simulink model "modelo_nlinear_iris"  (R2016a)
settings: Solver=ode1  StartTime=0.0  StopTime=25  FixedStep=0.01  RelTol=1e-3
undefined symbols (not defined in the file): Regions
settings Model: Creator=schul  LastModifiedBy=schul

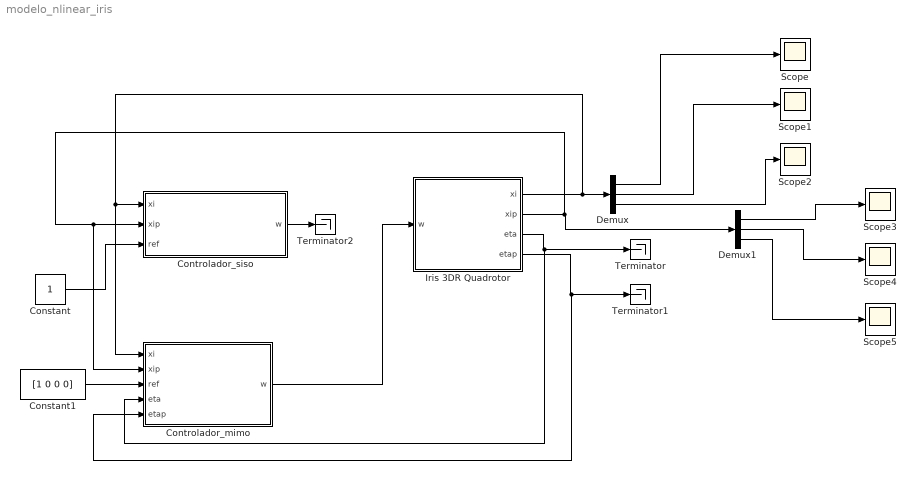
== system modelo_nlinear_iris ==
  Constant : Constant
  Constant1 : Constant  Value=[1 0 0 0]
  Controlador_mimo : Subsystem  mask{g=9.81, m=1.37, KT=15.67e-6, KD=2.551e-7, lx=0.13, ly=0.21, Ir=2.5206e-10, Ixx=0.0219, Iyy=0.0109, Izz=0.0306, Ax=0.25, Ay=0.25, Az=0.25}
  Controlador_siso : Subsystem  mask{g=9.81, m=1.37, KT=15.67e-6, KD=2.551e-7, lx=0.13, ly=0.21, Ir=2.5206e-10, Ixx=0.0219, Iyy=0.0109, Izz=0.0306, Ax=0.25, Ay=0.25, Az=0.25, Regions=Regions}
  Demux : Demux  Outputs=3
  Demux1 : Demux  Outputs=3
  Iris 3DR Quadrotor : Subsystem  mask{g=9.81, m=1.37, KT=15.67e-6, KD=2.551e-7, lx=0.13, ly=0.21, Ir=2.5206e-10, Ixx=0.0219, Iyy=0.0109, Izz=0.0306, Ax=0.25, Ay=0.25, Az=0.25}
  Scope{,1..5} (6 alike) : Scope
  Terminator : Terminator
  Terminator1 : Terminator
  Terminator2 : Terminator
  wires:
  Demux/1 -> Scope/1
  Demux/2 -> Scope1/1
  Demux/3 -> Scope2/1
  Demux1/1 -> Scope3/1
  Demux1/2 -> Scope4/1
  Demux1/3 -> Scope5/1
  Iris 3DR Quadrotor/1(xi) -> Controlador_mimo/1(xi), Controlador_siso/1(xi), Demux/1
  Iris 3DR Quadrotor/2(xip) -> Controlador_mimo/2(xip), Controlador_siso/2(xip), Demux1/1
  Constant/1 -> Controlador_siso/3(ref)
  Constant1/1 -> Controlador_mimo/3(ref)
  Iris 3DR Quadrotor/4(etap) -> Controlador_mimo/5(etap), Terminator1/1
  Iris 3DR Quadrotor/3(eta) -> Controlador_mimo/4(eta), Terminator/1
  Controlador_siso/1(w) -> Terminator2/1
  Controlador_mimo/1(w) -> Iris 3DR Quadrotor/1(w)

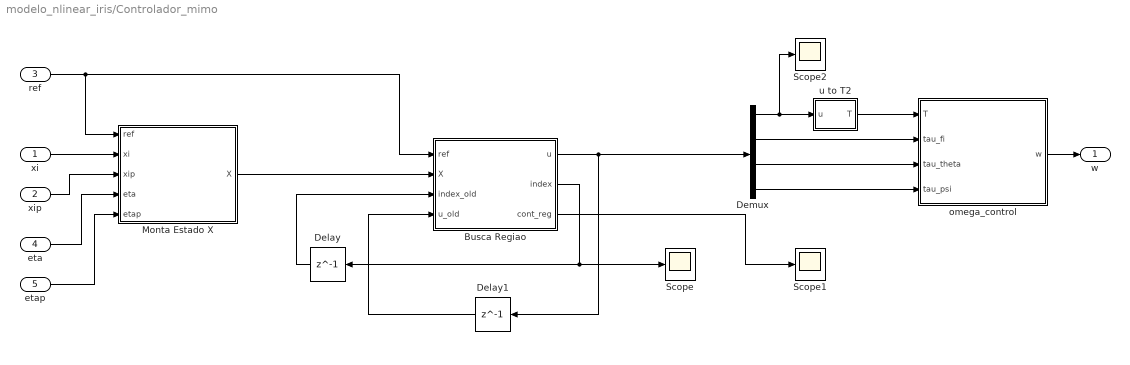
== system modelo_nlinear_iris/Controlador_mimo ==
  xi : Inport
  xip : Inport  Port=2
  ref : Inport  Port=3
  eta : Inport  Port=4
  etap : Inport  Port=5
  Busca Regiao : MATLAB Function  InitFcn=|  TreatAsAtomicUnit=on
      | hue = load('struct_regions.mat');
      | struct_regions = hue.reg_struct;
  Delay : Delay  DelayLength=1  InitialCondition=0
  Delay1 : Delay  DelayLength=1  InitialCondition=[0 0 0 0]'
  Demux : Demux
  Monta Estado X : MATLAB Function  TreatAsAtomicUnit=on
  Scope : Scope
  Scope1 : Scope
  Scope2 : Scope
  omega_control : MATLAB Function  TreatAsAtomicUnit=on
  u to T2 : MATLAB Function  TreatAsAtomicUnit=on
  w : Outport
  wires:
  Busca Regiao/2(index) -> Delay/1, Scope/1
  Delay/1 -> Busca Regiao/3(index_old)
  Delay1/1 -> Busca Regiao/4(u_old)
  omega_control/1(w) -> w/1
  Demux/4 -> omega_control/4(tau_psi)
  Demux/3 -> omega_control/3(tau_theta)
  Demux/2 -> omega_control/2(tau_fi)
  Demux/1 -> Scope2/1, u to T2/1(u)
  u to T2/1(T) -> omega_control/1(T)
  Busca Regiao/1(u) -> Delay1/1, Demux/1
  xi/1 -> Monta Estado X/2(xi)
  xip/1 -> Monta Estado X/3(xip)
  eta/1 -> Monta Estado X/4(eta)
  etap/1 -> Monta Estado X/5(etap)
  ref/1 -> Monta Estado X/1(ref), Busca Regiao/1(ref)
  Monta Estado X/1(X) -> Busca Regiao/2(X)
  Busca Regiao/3(cont_reg) -> Scope1/1

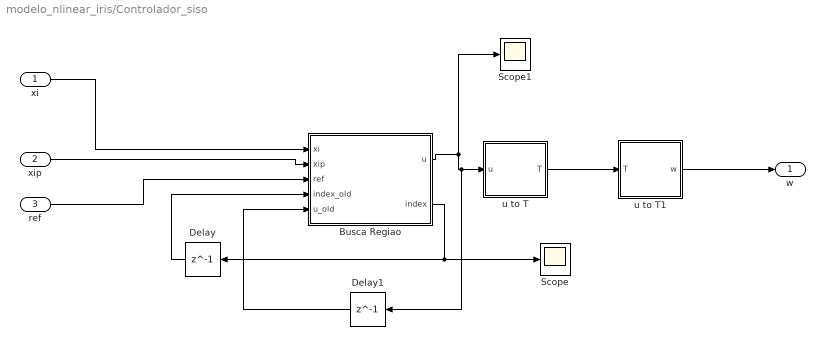
== system modelo_nlinear_iris/Controlador_siso ==
  xi : Inport
  xip : Inport  Port=2
  ref : Inport  Port=3
  Busca Regiao : MATLAB Function  TreatAsAtomicUnit=on
  Delay : Delay  DelayLength=1  InitialCondition=0
  Delay1 : Delay  DelayLength=1  InitialCondition=0
  Scope : Scope
  Scope1 : Scope
  u to T : MATLAB Function  TreatAsAtomicUnit=on
  u to T1 : MATLAB Function  TreatAsAtomicUnit=on
  w : Outport
  wires:
  Busca Regiao/2(index) -> Scope/1, Delay/1
  Delay/1 -> Busca Regiao/4(index_old)
  xi/1 -> Busca Regiao/1(xi)
  u to T1/1(w) -> w/1
  ref/1 -> Busca Regiao/3(ref)
  xip/1 -> Busca Regiao/2(xip)
  u to T/1(T) -> u to T1/1(T)
  Busca Regiao/1(u) -> Delay1/1, u to T/1(u), Scope1/1
  Delay1/1 -> Busca Regiao/5(u_old)

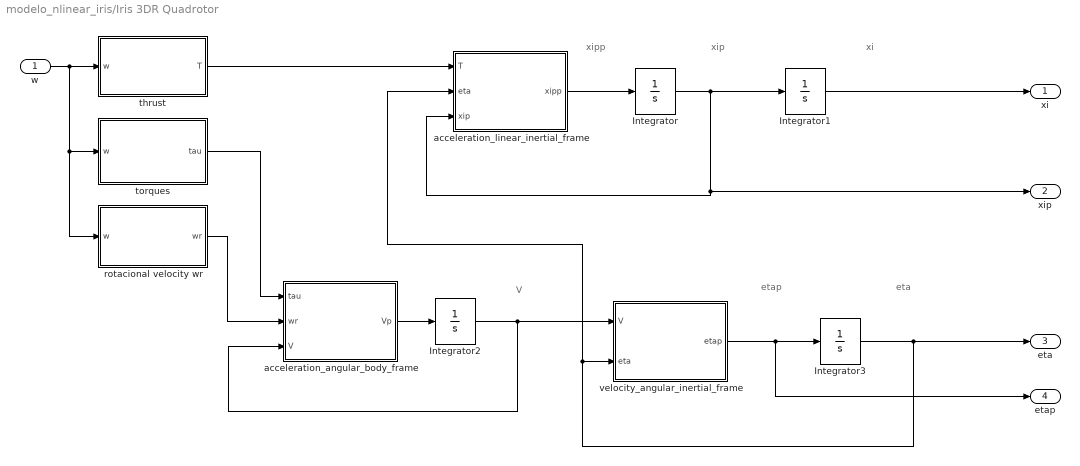
== system modelo_nlinear_iris/Iris 3DR Quadrotor ==
  note: xipp
  note: xip
  note: xi
  note: V
  note: etap
  note: eta
  w : Inport
  Integrator : Integrator  InitialCondition=[0 0 0]
  Integrator1 : Integrator  InitialCondition=[0 0 0]
  Integrator2 : Integrator  InitialCondition=[0 0 0]
  Integrator3 : Integrator  InitialCondition=[0 0 0 ]
  acceleration_angular_body_frame : MATLAB Function  TreatAsAtomicUnit=on
  acceleration_linear_inertial_frame : MATLAB Function  TreatAsAtomicUnit=on
  rotacional velocity wr : MATLAB Function  TreatAsAtomicUnit=on
  thrust : MATLAB Function  TreatAsAtomicUnit=on
  torques : MATLAB Function  TreatAsAtomicUnit=on
  velocity_angular_inertial_frame : MATLAB Function  TreatAsAtomicUnit=on
  xi : Outport
  xip : Outport  Port=2
  eta : Outport  Port=3
  etap : Outport  Port=4
  wires:
  w/1 -> rotacional velocity wr/1(w), torques/1(w), thrust/1(w)
  acceleration_angular_body_frame/1(Vp) -> Integrator2/1
  Integrator2/1 -> velocity_angular_inertial_frame/1(V), acceleration_angular_body_frame/3(V)
  rotacional velocity wr/1(wr) -> acceleration_angular_body_frame/2(wr)
  torques/1(tau) -> acceleration_angular_body_frame/1(tau)
  velocity_angular_inertial_frame/1(etap) -> etap/1, Integrator3/1
  acceleration_linear_inertial_frame/1(xipp) -> Integrator/1
  Integrator/1 -> acceleration_linear_inertial_frame/3(xip), xip/1, Integrator1/1
  Integrator3/1 -> eta/1, acceleration_linear_inertial_frame/2(eta), velocity_angular_inertial_frame/2(eta)
  thrust/1(T) -> acceleration_linear_inertial_frame/1(T)
  Integrator1/1 -> xi/1

== matlab function modelo_nlinear_iris/Iris 3DR Quadrotor/velocity_angular_inertial_frame ==
  data: V input; eta input; etap output double size=3
function etap = fcn(V, eta)
%Angular velocity at inertial frame
etap = [V(1) + V(2)*sin(eta(1))*tan(eta(2)) + V(3)*cos(eta(1))*tan(eta(2));
        V(2)*cos(eta(1)) - V(3)*sin(eta(1));
        V(2)*sin(eta(1))/cos(eta(2)) + V(3)*cos(eta(1))/cos(eta(2))];
    
% etap(1) = V(1) + V(2)*sin(eta(1))*tan(eta(2)) + V(3)*cos(eta(1))*tan(eta(2));
% etap(2) = V(2)*cos(eta(1)) - V(3)*sin(eta(1));
% etap(3) = V(2)*sin(eta(1))/cos(eta(2)) + V(3)*cos(eta(1))/cos(eta(2));

== matlab function modelo_nlinear_iris/Iris 3DR Quadrotor/acceleration_linear_inertial_frame ==
  data: T input; eta input; xipp output double size=3; xip input; g parameter; m parameter; Ax parameter; Ay parameter; Az parameter
function xipp = fcn(T, eta, xip, g, m, Ax, Ay, Az)
%Linear Acceleration at inertial frame
% xipp(1) = -Ax/m*xip(1) + 1/m*(cos(eta(1))*sin(eta(2))*cos(eta(6)) + sin(eta(3))*sin(eta(1)))*T;
% xipp(2) = -Ay/m*xip(2) + 1/m*(cos(eta(1))*sin(eta(2))*sin(eta(3)) - cos(eta(3))*sin(eta(1)))*T;
% xipp(3) = -Az/m*xip(3) - g + 1/m*(cos(eta(1))*cos(eta(2)))*T;

xipp = [-Ax/m*xip(1) + 1/m*(cos(eta(1))*sin(eta(2))*cos(eta(3)) + sin(eta(3))*sin(eta(1)))*T;
        -Ay/m*xip(2) + 1/m*(cos(eta(1))*sin(eta(2))*sin(eta(3)) - cos(eta(3))*sin(eta(1)))*T;
        -Az/m*xip(3) - g + 1/m*(cos(eta(1))*cos(eta(2)))*T];

== matlab function modelo_nlinear_iris/Iris 3DR Quadrotor/thrust ==
  data: w input; KT parameter; T output double size=1
function T  = fcn(w, KT)
%Calculate the Thrust force generated by the rotors
T = KT*(w(1)^2 + w(2)^2 + w(3)^2 + w(4)^2);

== matlab function modelo_nlinear_iris/Iris 3DR Quadrotor/torques ==
  data: w input double; tau output double size=3; lx parameter double size=1; ly parameter double size=1; KT parameter double size=1; KD parameter double size=1
function tau = fcn(w, lx, ly, KT, KD)
%Calculate the Torques generated by the rotors
% tau(1) = KT*ly*(-w(1)^2 + w(2)^2 + w(3)^2 - w(4)^2);
% tau(2) = KT*lx*(w(1)^2 - w(2)^2 + w(3)^2 -w(4)^2);
% tau(3) = KD(-w(1)^2 - w(2)^2 + w(3)^2 + w(4)^2);

tau = [KT*ly*(-w(1)^2 + w(2)^2 + w(3)^2 - w(4)^2);
       KT*lx*(w(1)^2 - w(2)^2 + w(3)^2 -w(4)^2);
       KD*(-w(1)^2 - w(2)^2 + w(3)^2 + w(4)^2)];

== matlab function modelo_nlinear_iris/Iris 3DR Quadrotor/acceleration_angular_body_frame ==
  data: tau input; wr input; V input double size=3; Vp output double size=3; Ixx parameter; Iyy parameter; Izz parameter; Ir parameter
function Vp = fcn(tau, wr, V, Ixx, Iyy, Izz, Ir)
%Angular acceleration at body frame
Vp = [(Iyy - Izz)/Ixx*V(2)*V(3) - Ir*V(2)*wr/Ixx + tau(1)/Ixx;
     (Izz - Ixx)/Iyy*V(1)*V(3) + Ir*V(1)*wr/Iyy + tau(2)/Iyy;
     (Ixx - Iyy)/Izz*V(1)*V(2) + tau(3)/Izz];

% Vp(1) = (Iyy - Izz)/Ixx*V(2)*V(3) - Ir*V(2)*wr/Ixx + tau(1)/Ixx;
% Vp(2) = (Izz - Ixx)/Iyy*V(1)*V(3) + Ir*V(1)*wr/Iyy + tau(2)/Iyy;
% Vp(3) = (Ixx - Iyy)/Izz*V(1)*V(2) + tau(3)/Izz;

== matlab function modelo_nlinear_iris/Controlador_siso/Busca Regiao ==
  data: xi input; u output double size=1; xip input; ref input; index_old input; index output; u_old input
function [u, index] = fcn(xi, xip, ref, index_old, u_old)
Regions = cell(34, 4);
Regions{1,1} = ...
  [-4.7678193579478347E-5 -0.0043030705370811235 0.0043030705370811235;
   0.35454713969010543 31.926731615246421 -31.926731615246421;
   1 0 0;
   -1 0 0;
   0 -1 0;
   0 0 1;
   0 0 -1];
Regions{2,1} = ...
  [-3.5576487707234271E-5 -0.0032036388047997572 0.0032036388047997572;
   0.23261867147448964 20.940966847397387 -20.940966847397387;
   1 0 0;
   -1 0 0;
   0 -1 0;
   0 0 1;
   0 0 -1];
Regions{3,1} = ...
  [-2.3313238553360363E-5 -0.0020987212787212791 0.0020987212787212791;
   0.11097681558999362 9.99000999000999 -9.99000999000999;
   1 0 0;
   -1 0 0;
   0 -1 0;
   0 0 1;
   0 0 -1];
Regions{4,1} = ...
  [-1.1108779240558364E-5 -0.0010000000000000002 0.0010000000000000002;
   1 0 0;
   0 1 0;
   0.01 1 0;
   0.0109982 1 0;
   0.011097840324 1 0;
   0.01110778642114168 1 0;
   -1 0 0;
   0 -1 0;
   0 0 1;
   0 0 -1];
Regions{5,1} = ...
  [-0.4745723890284354 -42.831288512143423 42.831288512143423;
   0.4745723890284354 42.831288512143423 -42.831288512143423;
   1 -0 -0;
   -1 -0 -0;
   -0 -1 -0;
   -0.01 -1 -0;
   -0.010950742761097157 -0.99571687114878571 -0.0042831288512143427;
   -0.011010358919756659 -0.99211179411683148 -0.0078882058831685215;
   -0.0109932399356526 -0.98967515026796271 -0.010324849732037338;
   -0.010980550568091243 -0.98844348099797064 -0.011556519002029395;
   -0 -0 1;
   -0 -0 -1];
Regions{6,1} = ...
  [23.694126938983068 2132.8898915901432 24.936967095489916;
   -1 0 0;
   0 -1 0;
   -0.0083489088688396516 -0.76150586929657549 -0.0015448196353382284;
   -0.0026577290318065827 -0.23933195366754667 -0.0015521120123234578;
   0 0 -1];
Regions{7,1} = ...
  [-3.5736117010237933 -322.60541387854028 9.0126256048592666;
   35.9203876604541 3234.6775959430288 20.977482846401614;
   -36.007729550648484 -3241.7630562380486 9.891548739137896;
   -35.575824110941262 -3202.7726479893631 -0.98737439514076542;
   -1 0 0;
   0 -1 0;
   -0.01 -1 0;
   -0.0073974270449351526 -0.67582369437619516 -0.00098915487391378933;
   -0.0035800558014664526 -0.32318715074989068 -0.00098915487391378846;
   0 0 -1];
Regions{8,1} = ...
  [-3.4393645363778958E-14 -4.4488331783609624E-12 10.000000000000002;
   55.908433100960636 5047.0965255315332 15.447272936931789;
   -55.509270630682252 -5002.2516760820145 4.5033521640331742;
   -49.928197214962971 -4498.4235616114711 -4.9528767770469067;
   0 -1 0;
   -0.01 -1 0;
   -0.0054472729369317756 -0.49977483239179848 -0.0004503352164033172;
   0 0 -1];
Regions{9,1} = ...
  [-1.4210854715202004E-14 -1.8189894035458565E-12 10;
   -9.9819999999999709 -998.20000000000437 10;
   120.96040324000003 11097.840324 10.000000000000014;
   -109.98200000000001 -9999.9999999999982 7.1054273576010019E-15;
   0 0 -1];
Regions{10,1} = ...
  [-2.8421709430404007E-14 -3.637978807091713E-12 9.9999999999999858;
   92.653637590158226 8357.7606966965341 19.092396937680718;
   0.0091657234350158243 0.8258120372696538 0.00090923969376807256;
   -100.90596937680712 -9092.3969376807145 -1.4210854715202004E-14;
   0 0 -1];
Regions{11,1} = ...
  [-2.8421709430404007E-14 -5.4569682106375694E-12 10.000000000000014;
   0.01232621136628336 1.1107840324 -0.00099999999999999915;
   -110.97840323999989 -9999.99999999999 1.0658141036401503E-14;
   -0.010998200000000007 -1.0000000000000007 1.7347234759768071E-18;
   0 0 -1];
Regions{12,1} = ...
  [0.44871546871033335 44.871546871033992 9.5504753869862036;
   -5.4374678456452763 -543.746784564528 15.447272936931784;
   115.52293539435468 10554.093539435467 15.447272936931769;
   -109.98199999999997 -9999.9999999999982 1.4210854715202004E-14;
   0.00044952461301378359 0.044952461301378421 -0.0004503352164033211;
   0 0 -1];
Regions{13,1} = ...
  [-4.981225344014157 -449.32816977724769 8.9735585781895537;
   0.0054931253187936319 0.4945277295094152 0.00015245665911104293;
   -55.533020004124182 -4999.5597558570826 9.34964219633153;
   -1 0 0;
   0 0 -1];
Regions{14,1} = ...
  [-11.077864211415928 -998.19999999992069 9.9999999999997584;
   0.012338242742582391 1.1107840323999991 -0.00099999999999999482;
   0.012472065092588608 1.1228424945141671 -0.002099819999999997;
   -111.07786421141728 -10000.000000000044 1.1013412404281553E-13;
   -1 0 0;
   0 0 -1];
Regions{15,1} = ...
  [-5.5315204172872328 -498.8752376934911 9.5504753869862;
   0.0056231965375380345 0.50625437984684651 -0.0015447272936931779;
   -55.563452155174872 -5002.2516760820163 4.5033521640331884;
   -1 0 0];
Regions{16,1} = ...
  [-3.2147352074608762 -321.47352074608762 19.957952560598528;
   113.56379145036549 10358.179145036549 21.012994350765105;
   -109.98199999999999 -9999.9999999999982 7.1054273576010019E-15;
   0.00035042011291057558 0.035042011291057329 -0.000995506599833093];
Regions{17,1} = ...
  [32.234103853173529 2901.9007827876403 30.274266774760921;
   -35.882628913025989 -3230.4696795779287 9.5760457398899845;
   -35.4837549242375 -3194.4611635397459 -1.2195722887359572;
   -1 0 0;
   0 -1 0;
   -0.0074099371086974019 -0.67695303204220714 -0.00095760457398899861;
   -0.0036030215384638244 -0.32526036734668562 -0.00093123543369098491;
   0.00035929431565380303 0.032435054813732322 -0.00090613794106790026];
Regions{18,1} = ...
  [-5.437467845645287 -498.87523769349173 20.537688174198991;
   55.908433100960622 5047.0965255315332 14.450070139729007;
   -55.509270630682266 -5002.2516760820172 4.50335216403316;
   -49.928197214963014 -4498.4235616114756 -4.9528767770469493;
   0 -1 0;
   -0.01 -1 0;
   -0.005447272936931773 -0.49977483239179832 -0.00045033521640331546;
   -3.4694469519536142E-18 -3.3306690738754696E-16 -0.000999000999001005 ...
   ];
Regions{19,1} = ...
  [7.28920794240582E-15 4.1723781794201095E-13 20.987212787212773;
   -9.9819999999999958 -998.19999999999823 9.0027972027972289;
   120.96040323999996 11097.840323999997 9.99999999999998;
   -109.982 -10000 0;
   0 0 -1];
Regions{20,1} = ...
  [92.65363759015824 8357.76069669654 18.095194140477947;
   0.0091657234350158278 0.82581203726965391 0.00090923969376807223;
   -100.90596937680714 -9092.3969376807145 7.1054273576010019E-15;
   3.4694469519536142E-18 4.4408920985006262E-16 -0.0009990009990010016 ...
   ;
   0 0 -1];
Regions{21,1} = ...
  [-10.978403240000031 -998.20000000000232 20.987212787212762;
   123.05267069141681 11097.840324000004 9.0027972027972236;
   0.012326211366283361 1.1107840324000002 -0.000999999999999999;
   -110.97840324 -10000 -1.0658141036401503E-14;
   -1.7347234759768071E-18 0 -0.00099900099900099987];
Regions{22,1} = ...
  [-4.9667187833788873 -496.6718783378883 25.466712082953503;
   115.49845125504395 10551.645125504396 14.926151678218261;
   -109.98200000000001 -10000 0;
   0.000451548757994703 0.045154875799470306 -0.00040725324538181187;
   0 0 -1];
Regions{23,1} = ...
  [0.0054733298775250429 0.49274209469451241 0.00018811767412981947;
   -55.288458109229587 -4977.499210300296 8.9090697792521;
   -0.0050171051242307108 -0.45256468185275278 -0.00097983731246170571;
   0.00050030712637432959 0.045129876665875535 -0.00090129134812195685;
   0 0 -1];
Regions{24,1} = ...
  [111.09003569654867 10001.09674358042 20.98721278721279;
   0.012227773970795832 1.1008299540783222 -0.00090027972027971991;
   0.012350569328002306 1.11189480009442 -0.0019901456419580406;
   -111.0778642114168 -10000 -7.1054273576010019E-15;
   -1 0 0;
   -0.011097840324000005 -1.0000000000000004 -5.2041704279304213E-18;
   0.0011066797414002755 0.0997202797202793 -0.00099900099900100334;
   0 0 -1];
Regions{25,1} = ...
  [50.2486064642674 4523.724663609547 25.466712082953503;
   0.0055930138213312166 0.50353226936256545 -0.0014926151678218268;
   -55.313926563341845 -4979.7475308297862 4.0725324538181233;
   -1 0 0;
   -0.0055664476676658145 -0.50202524691702133 -0.00040725324538181274;
   0.00055508771846793023 0.050062098049207582 -0.00095838959145453685];
Regions{26,1} = ...
  [50.210276704433106 4524.3037095686823 35.972396811218772;
   -55.264284804103887 -4979.774786850624 3.5780239310773041;
   0 -1 0;
   -0.0054717715195896121 -0.50202252131493763 -0.00035780239310773034;
   0.00054498868245701423 0.050001465060386052 -0.0020584595507509296];
Regions{27,1} = ...
  [-9.9819999999999851 -998.19999999999709 32.0363880479976;
   120.96040323999996 11097.840323999995 7.9096726892927762;
   -109.982 -10000 -7.1054273576010019E-15;
   3.4694469519536142E-18 2.2204460492503131E-16 -0.0020940966847397356 ...
   ;
   5.2041704279304213E-18 5.5511151231257827E-16 -0.003299829586224233];
Regions{28,1} = ...
  [-9.9819999999999869 -998.19999999999732 15.471825866013484;
   120.96040323999999 11097.840323999995 9.54844920873671;
   -6.97196518640781E-15 -9.8208701849860536E-13 14.975201274766293;
   -109.98199999999997 -9999.9999999999982 7.1054273576010019E-15;
   0 0 -1];
Regions{29,1} = ...
  [111.00380784680635 10002.30988769129 32.0363880479976;
   0.012216866422039452 1.1008419560380582 -0.00079096726892927821;
   -110.97840324000002 -10000.000000000002 -2.4868995751603507E-14;
   -0.0109982 -1 8.6736173798840355E-19;
   0.001095421200600178 0.099600043698075624 -0.0020940966847397356;
   0 0 -1];
Regions{30,1} = ...
  [110.01727982353762 10003.527982353762 43.030705370811226;
   -109.98199999999999 -9999.9999999999982 7.1054273576010019E-15;
   -0.01 -1 0;
   0.00099478328988248516 0.099478328988248488 -0.0031926731615246435;
   0.0011003624833158913 0.11003624833158898 -0.0068313502743594977];
Regions{31,1} = ...
  [4.7678193579478347E-5 0.0043030705370811235 -0.0043030705370811235;
   -0.35454713969010543 -31.926731615246421 31.926731615246421;
   1 0 0;
   -1 0 0;
   0 -1 0;
   -0.01 -1 0;
   -0.0109982 -1 0;
   -0.011062385610030988 -0.99680732683847539 -0.0031926731615246435;
   -0.011045612794563585 -0.99440192553361717 -0.0055980744663829034;
   0 0 1];
Regions{32,1} = ...
  [3.5576487707234271E-5 0.0032036388047997572 -0.0032036388047997572;
   -0.23261867147448964 -20.940966847397387 20.940966847397387;
   1 0 0;
   -1 0 0;
   0 -1 0;
   -0.01 -1 0;
   -0.0109982 -1 8.6736173798840355E-19;
   -0.011097840324 -1 1.7347234759768071E-18;
   -0.011084524553994231 -0.9979059033152603 -0.0020940966847397373;
   0 0 1];
Regions{33,1} = ...
  [2.3313238553360363E-5 0.0020987212787212791 -0.0020987212787212791;
   -0.11097681558999362 -9.99000999000999 9.99000999000999;
   1 0 0;
   -1 0 0;
   0 -1 0;
   -0.01 -1 0;
   -0.0109982 -1 -8.6736173798840355E-19;
   -0.011097840324 -1 0;
   -0.01110778642114168 -1 0;
   0 0 1];
Regions{34,1} = ...
  [1.1108779240558364E-5 0.0010000000000000002 -0.0010000000000000002;
   1 0 0;
   -1 0 0;
   0 -1 0;
   -0.01 -1 0;
   -0.0109982 -1 0;
   -0.011097840324 -1 0;
   -0.01110778642114168 -1 0;
   0 0 1];
Regions{1,2} = [-0.000985567407265781; 9.8446719163398377; 500; 500; 1; ...
                11; 1];
Regions{2,2} = [-0.00098784846979599827; 9.8555099481016253; 500; 500; ...
                1; 11; 1];
Regions{3,2} = [-0.0009877274813269092; 9.842540413623361; 500; 500; 1; ...
                11; 1];
Regions{4,2} = [-0.00098523829540369872; 500; 50; 50; 50.000981; 50.00205992342; ...
                50.003148621555788; 500; 1; 11; 1];
Regions{5,2} = [19.62; 9.81; 500; 500; 1; 1; 1; 1; 1; 1; 11; 1];
Regions{6,2} = [-2157.8268586856329; 500; 1; 0.76305068893191363; 0.24088406567987009; ...
                1];
Regions{7,2} = [313.59278827368144; -3255.6550787894303; 3251.4915074989103; ...
                3223.3800223845037; 500; 1; 1; 0.67681284925010887; 0.32417630562380439; ...
                1];
Regions{8,2} = [-9.9999999999967031; -5062.543798468465; 5017.3683239179818; ...
                4522.996438388519; 1; 1; 0.50022516760820179; 1];
Regions{9,2} = [-9.9999999999989218; 988.20000000000073; -11107.840324; ...
                10019.62; 1];
Regions{10,2} = [-9.9999999999968132; -8391.2926478799691; -0.830323079227997; ...
                 9129.8562204724421; 1];
Regions{11,2} = [-9.9999999999955538; -1.1141407869431375; 10041.198468399991; ...
                 1.0019620000000005; 1];
Regions{12,2} = [-54.422022258019751; 528.29951162759517; -10569.5408123724; ...
                 10019.619999999997; -0.044502126084974947; 1];
Regions{13,2} = [441.130907472318; -0.497709634437065; 5020.5982745753809; ...
                 500; 1];
Regions{14,2} = [992.31243111560821; -1.1165591896132012; -1.1275674991129947; ...
                 10062.972431115733; 500; 1];
Regions{15,2} = [490.39159349782096; -0.50777363679885; 5028.2592428157232; ...
                 500];
Regions{16,2} = [301.515568185489; -10379.192139387314; 10019.619999999999; ...
                 -0.034046504691224388];
Regions{17,2} = [-2932.175049562401; 3240.5136338380385; 3215.3007358284817; ...
                 500; 1; 0.67791063661619611; 0.32619160278037662; -0.031528916872664459; ...
                 ];
Regions{18,2} = [478.33754951929404; -5061.5465956712633; 5017.3683239179836; ...
                 4522.9964383885226; 1; 1; 0.50022516760820168; 0.00099900099900129824; ...
                 ];
Regions{19,2} = [-20.987212787213252; 989.19720279720059; -11107.840323999995; ...
                 10019.619999999999; 1];
Regions{20,2} = [-8390.2954450827674; -0.8303230792279972; 9129.856220472444; ...
                 0.000999000999000632; 1];
Regions{21,2} = [979.17125561278942; -11130.575552318489; -1.1141407869431377; ...
                 10041.1984684; 0.0009990009990010762];
Regions{22,2} = [471.20516625493474; -10566.571277182615; 10019.62; -0.044747622554088373; ...
                 1];
Regions{23,2} = [-0.49595657562772588; 4998.940187824167; 0.45432640710272243; ...
                 -0.044306555401591785; 1];
Regions{24,2} = [-10065.440905898895; -1.106663822293126; -1.1166843762270287; ...
                 10062.972431115688; 500; 1.0041198468400006; -0.099132111000567846; ...
                 1];
Regions{25,2} = [-4559.041393707801; -0.5050978172808569; 5006.1377927682706; ...
                 500; 0.50350606756317284; -0.049210764899256354];
Regions{26,2} = [-4560.2761063799007; 4995.8167629195468; 1; 0.50238032370804531; ...
                 -0.047943005509635261];
Regions{27,2} = [966.163611951999; -11105.749996689288; 10019.62; 0.0020940966847393661; ...
                 0.0032998295862236571];
Regions{28,2} = [982.72817413398388; -11107.388773208733; -14.975201274764913; ...
                 10019.619999999999; 1];
Regions{29,2} = [-10055.929276138939; -1.1043882369584446; 10041.198468400002; ...
                 1.001962; -0.09770136229907167; 1];
Regions{30,2} = [-10046.558687724573; 10019.619999999999; 1; -0.096285655826723771; ...
                 -0.10320489805722954];
Regions{31,2} = [-0.0019711348145315618; 19.689343832679675; 500; 500; ...
                 1; 1; 1.001962; 1.002150912456732; 1.0021652239270329; ...
                 11];
Regions{32,2} = [-0.0019756969395919965; 19.711019896203251; 500; 500; ...
                 1; 1; 1.001962; 1.00411984684; 1.0043261411219484; 11];
Regions{33,2} = [-0.0019754549626538184; 19.685080827246722; 500; 500; ...
                 1; 1; 1.001962; 1.00411984684; 1.0062972431115689; 11];
Regions{34,2} = [-0.0019704765908073974; 500; 500; 1; 1; 1.001962; 1.00411984684; ...
                 1.0062972431115689; 11];
Regions{1,3} = [0 0 0];
Regions{2,3} = [1.1102230246251565E-16 7.1054273576010019E-15 -7.1054273576010019E-15 ...
                ];
Regions{3,3} = [-5.5511151231257827E-17 -7.1054273576010019E-15 7.1054273576010019E-15 ...
                ];
Regions{4,3} = [0 0 0];
Regions{5,3} = [-0.4745723890284354 -42.831288512143423 42.831288512143423 ...
                ];
Regions{6,3} = [-26.492911311603478 -2384.9413070342462 15.448196353382283 ...
                ];
Regions{7,3} = [-36.007729550648484 -3241.7630562380486 9.891548739137896 ...
                ];
Regions{8,3} = [-55.509270630682252 -5002.2516760820145 4.5033521640331742 ...
                ];
Regions{9,3} = [-109.98200000000001 -9999.9999999999982 7.1054273576010019E-15 ...
                ];
Regions{10,3} = [-100.90596937680712 -9092.3969376807145 -1.4210854715202004E-14 ...
                 ];
Regions{11,3} = [5.6565863104651726E-14 5.1016968427575193E-12 -1.4210854715202004E-14 ...
                 ];
Regions{12,3} = [-109.98199999999997 -9999.9999999999982 1.4210854715202004E-14 ...
                 ];
Regions{13,3} = [-55.533020004124182 -4999.5597558570826 9.34964219633153 ...
                 ];
Regions{14,3} = [-5.4439786012494551E-13 -4.9013237912731711E-11 1.2789769243681803E-13 ...
                 ];
Regions{15,3} = [-1.9095836023552692E-14 -1.7195134205394424E-12 2.8421709430404007E-14 ...
                 ];
Regions{16,3} = [-109.98199999999999 -9999.9999999999982 7.1054273576010019E-15 ...
                 ];
Regions{17,3} = [-35.882628913025989 -3230.4696795779287 9.5760457398899845 ...
                 ];
Regions{18,3} = [-55.509270630682266 -5002.2516760820172 4.50335216403316 ...
                 ];
Regions{19,3} = [-109.982 -10000 0];
Regions{20,3} = [-100.90596937680714 -9092.3969376807145 7.1054273576010019E-15 ...
                 ];
Regions{21,3} = [2.4424906541753444E-14 2.2026824808563106E-12 7.1054273576010019E-15 ...
                 ];
Regions{22,3} = [-109.98200000000001 -10000 0];
Regions{23,3} = [-55.288458109229587 -4977.499210300296 8.9090697792521 ...
                 ];
Regions{24,3} = [3.1641356201816961E-14 2.8492763703980017E-12 2.8421709430404007E-14 ...
                 ];
Regions{25,3} = [0 0 0];
Regions{26,3} = [-55.264284804103887 -4979.774786850624 3.5780239310773041 ...
                 ];
Regions{27,3} = [-109.982 -10000 -7.1054273576010019E-15];
Regions{28,3} = [-109.98199999999997 -9999.9999999999982 7.1054273576010019E-15 ...
                 ];
Regions{29,3} = [1.1102230246251565E-16 7.1054273576010019E-15 -7.1054273576010019E-15 ...
                 ];
Regions{30,3} = [-109.98199999999999 -9999.9999999999982 7.1054273576010019E-15 ...
                 ];
Regions{31,3} = [0 0 0];
Regions{32,3} = [1.1102230246251565E-16 7.1054273576010019E-15 -7.1054273576010019E-15 ...
                 ];
Regions{33,3} = [-5.5511151231257827E-17 -7.1054273576010019E-15 7.1054273576010019E-15 ...
                 ];
Regions{34,3} = [0 0 0];
Regions{1,4} = -9.81;
Regions{2,4} = -9.8100000000000023;
Regions{3,4} = -9.8099999999999987;
Regions{4,4} = -9.81;
Regions{5,4} = 0;
Regions{6,4} = -2369.4931106808635;
Regions{7,4} = -3231.8715074989104;
Regions{8,4} = -4997.7483239179819;
Regions{9,4} = -10000;
Regions{10,4} = -9110.2362204724413;
Regions{11,4} = 19.62000000000511;
Regions{12,4} = -9999.9999999999964;
Regions{13,4} = -5000.978274575381;
Regions{14,4} = 19.619999999950821;
Regions{15,4} = 19.619999999998289;
Regions{16,4} = -9999.9999999999982;
Regions{17,4} = -3220.8936338380386;
Regions{18,4} = -4997.7483239179837;
Regions{19,4} = -9999.9999999999982;
Regions{20,4} = -9110.2362204724432;
Regions{21,4} = 19.620000000002214;
Regions{22,4} = -10000;
Regions{23,4} = -4979.3201878241671;
Regions{24,4} = 19.620000000002879;
Regions{25,4} = 19.62;
Regions{26,4} = -4976.1967629195469;
Regions{27,4} = -10000;
Regions{28,4} = -9999.9999999999982;
Regions{29,4} = 19.620000000000005;
Regions{30,4} = -9999.9999999999982;
Regions{31,4} = 19.62;
Regions{32,4} = 19.620000000000005;
Regions{33,4} = 19.619999999999997;
Regions{34,4} = 19.62;
    z = xi(3);
    zp = xip(3);
    index = index_old;
    u = u_old;
    for j = 1:size(Regions,1)
            A_CRi = Regions{j,1};
            b_CRi = Regions{j,2};
            flag = 0;
            for k = 1:size(A_CRi,1)
                %if(A_CRi(k,:)*[x(:,i); ref] > b_CRi(k))
                if(A_CRi(k,:)*[zp; z; ref]) > b_CRi(k)
    %                 if flag == 0 
    %                     cont_out = cont_out + 1;
    %                 end
                    flag = 1;
                end
            end
            if flag == 0        
                index = j;
            end
    end
    u_calc = double(Regions{index,3}*[zp; z; ref] + Regions{index,4});
    u = u_calc(1,1);

== matlab function modelo_nlinear_iris/Iris 3DR Quadrotor/rotacional velocity wr ==
  data: w input; wr output double size=1
function wr = fcn(w)
%Calculate the Torques generated by the rotors
wr = w(1)+w(3)-w(2)-w(4);

== matlab function modelo_nlinear_iris/Controlador_siso/u to T ==
  data: u input; T output; g parameter; m parameter
function T = fcn(u,g,m)

T = m*(u + g);

== matlab function modelo_nlinear_iris/Controlador_siso/u to T1 ==
  data: w output double; T input; KT parameter
function w = fcn(T, KT)

w1 = (T/(4*KT));
if w1 > 0
    w1 = w1^(1/2);
else
    w1 = 0;
end

w2 = (T/(4*KT));
if w2 > 0
    w2 = w2^(1/2);
else
    w2 = 0;
end

w3 = (T/(4*KT));
if w3 > 0
    w3 = w3^(1/2);
else
    w3 = 0;
end

w4 = (T/(4*KT));
if w4 > 0
    w4 = w4^(1/2);
else
    w1 = 0;
end
w = [w1 w2 w3 w4]

== matlab function modelo_nlinear_iris/Controlador_mimo/Busca Regiao ==
  data: ref input; X input; u output double size=4; index_old input; index output; u_old input double size=4; cont_reg output; struct_regions parameter
function [u, index, cont_reg] = fcn(ref, X, index_old, u_old,struct_regions)
                    
%     z = xi(3);
%     zp = xip(3);
    index = 0;%index_old;
    u = u_old;
    cont_reg = 0;
%     for j = 1:size(Regions,1)
%             A_CRi = Regions{j,1};
%             b_CRi = Regions{j,2};
%             flag = 0;
%             for k = 1:size(A_CRi,1)
%                 if(A_CRi(k,:)*[X; ref] > b_CRi(k))
%                 %if(A_CRi(k,:)*[zp; z; ref]) > b_CRi(k)
%     %                 if flag == 0 
%     %                     cont_out = cont_out + 1;
%     %                 end
%                     flag = 1;
%                 end
%             end
%             if flag == 0
%                 cont_reg = cont_reg + 1;        
%                 index = j;
%             end
%     end
%     if index == 0
%         index = index_old;
%     end
%     u_calc = double(Regions{index,3}*[X; ref] + Regions{index,4})
%     u = u_calc(1:4,1);

    
     for j = 1:size(struct_regions,2)
            A_CRi =  struct_regions(j).A;
            b_CRi =  struct_regions(j).b;
            flag = 0;
            for k = 1:size(A_CRi,1)
                if(A_CRi(k,:)*[X; ref] > b_CRi(k))
                %if(A_CRi(k,:)*[zp; z; ref]) > b_CRi(k)
    %                 if flag == 0 
    %                     cont_out = cont_out + 1;
    %                 end
                    flag = 1;
                end
            end
            if flag == 0
                cont_reg = cont_reg + 1;        
                index = j;
            end
    end
    if index == 0
        index = index_old;
    end
    u_calc = double(struct_regions(index).Kx*[X; ref] + struct_regions(index).Kc)
    u = u_calc(1:4,1);

%     [ u, index, cont_reg] = test_struct(X, ref, index_old);

end

== matlab function modelo_nlinear_iris/Controlador_mimo/Monta Estado X ==
  data: ref input; xi input; X output; xip input; eta input; etap input
function X = fcn(ref, xi, xip, eta, etap)
%#codegen
X = [xi(3);
    xip(3);
    eta(1);
    etap(1);
    eta(2);
    etap(2);
    eta(3);
    etap(3)];

== matlab function modelo_nlinear_iris/Controlador_mimo/omega_control ==
  data: T input; tau_fi input; tau_theta input; tau_psi input; w output; KT parameter; KD parameter; lx parameter; ly parameter
function w = fcn(T, tau_fi, tau_theta, tau_psi, KT, KD, lx, ly)

%Caso se queira incluir controle em psi, adicionar: [-tau_psi/(4KD),
%-tau_psi/(4KD), tau_psi/(4KD), tau_psi/(4KD)], respectivamente.

w1 = (T/(4*KT)-tau_fi/(4*KT*ly)-tau_theta/(4*KT*lx)-tau_psi/(4*KD));
if w1 > 0
    w1 = w1^(1/2);
else
    w1 = 0;
end

w2 = (T/(4*KT)+tau_fi/(4*KT*ly)+tau_theta/(4*KT*lx)-tau_psi/(4*KD));
if w2 > 0
    w2 = w2^(1/2);
else
    w2 = 0;
end

w3 = (T/(4*KT)+tau_fi/(4*KT*ly)-tau_theta/(4*KT*lx)+tau_psi/(4*KD));
if w3 > 0
    w3 = w3^(1/2);
else
    w3 = 0;
end

w4 = (T/(4*KT)-tau_fi/(4*KT*ly)+tau_theta/(4*KT*lx)+tau_psi/(4*KD));
if w4 > 0
    w4 = w4^(1/2);
else
    w4 = 0;
end

w = [w1;w2;w3;w4];

== matlab function modelo_nlinear_iris/Controlador_mimo/u to T2 ==
  data: u input; T output; g parameter; m parameter
function T = fcn(u,g,m)

T = u + m*g;
